simulink model "model2"  (R2020a)
settings: Solver=VariableStepAuto  StartTime=0.0  StopTime=50  RelTol=1e-3
libraries: SignalEditorBlockLib x1
settings Model: Creator=MILAD  LastModifiedBy=payagostar
settings DataIOCC: ReturnWorkspaceOutputs=off
settings DebuggingCC: ArithmeticOperatorsInVariantConditions=warning
settings SFSimCC: CustomCodeUndefinedFunction=UseInterfaceOnly

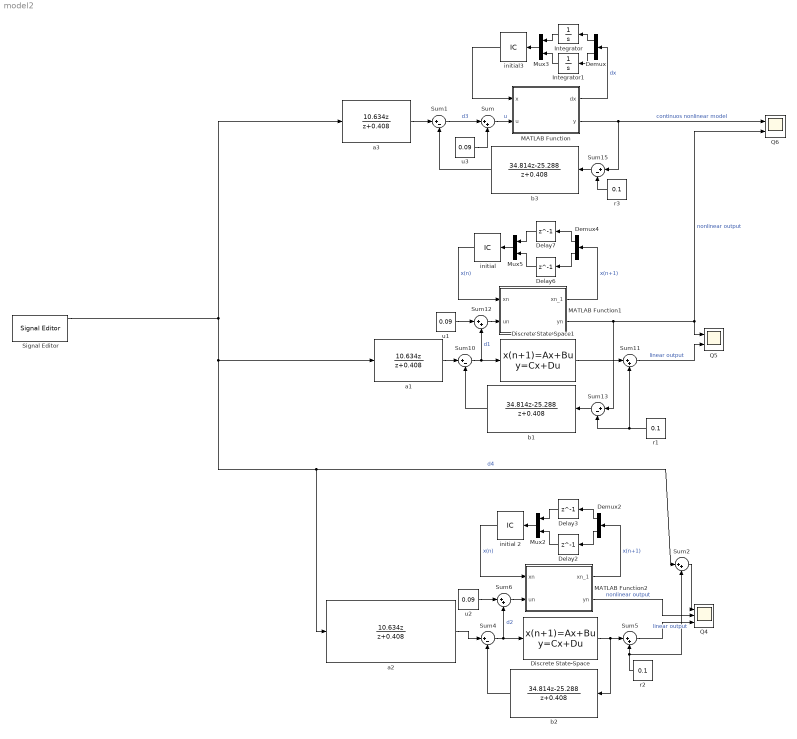
== system model2 ==
  " Q4" : Scope  NumInputPorts=3
  Delay{2..3,6..7} (4 alike) : Delay  DelayLength=1  InitialCondition=0  SampleTime=0.166
  Demux : Demux  Outputs=2
  Demux2 : Demux  Outputs=2
  Demux4 : Demux  Outputs=2
  Discrete State-Space : DiscreteStateSpace  A=[0.9884 0.1523;-0.1354 0.8361]  B=[0.01447;0.1693]  C=[1 0]  D=0  SampleTime=0.166
  Discrete State-Space1 : DiscreteStateSpace  A=[0.9884 0.1523;-0.1354 0.8361]  B=[0.01447;0.1693]  C=[1 0]  D=0  SampleTime=0.166
  Integrator : Integrator  InitialCondition=0.1
  Integrator1 : Integrator
  MATLAB Function : MATLAB Function  TreatAsAtomicUnit=on
  MATLAB Function1 : MATLAB Function  TreatAsAtomicUnit=on
  MATLAB Function2 : MATLAB Function  TreatAsAtomicUnit=on
  Mux2 : Mux  Inputs=2
  Mux3 : Mux  Inputs=2
  Mux5 : Mux  Inputs=2
  Q5 : Scope  NumInputPorts=2
  Q6 : Scope  NumInputPorts=2
  Signal Editor : SignalEditorBlockLib/Signal Editor  FileName=r.mat  ActiveScenario=Scenario  ActiveSignal=Signal 3  IsBus=off  OutputBusObjectStr=Bus: BusObject  SampleTime=0.166  Interpolate=off  ZeroCross=off  OutputAfterFinalValue=Setting to zero  Unit=inherit  PreserveSignalName=on
  Sum{,2,5..6,11..12} (6 alike) : Sum  Inputs=|++
  Sum{1,4,10,13,15} (5 alike) : Sum  Inputs=|+-
  a1 : DiscreteTransferFcn  Numerator=[10.634 0]  Denominator=[1, 0.408]  SampleTime=0.166
  a2 : DiscreteTransferFcn  Numerator=[10.634 0]  Denominator=[1 0.408]  SampleTime=0.166
  a3 : DiscreteTransferFcn  Numerator=[10.634 0]  Denominator=[1, 0.408]  SampleTime=0.166
  b1 : DiscreteTransferFcn  Numerator=[34.814 -25.288]  Denominator=[1, 0.408]  SampleTime=0.166
  b2 : DiscreteTransferFcn  Numerator=[34.814, -25.288]  Denominator=[1, 0.408]  SampleTime=0.166
  b3 : DiscreteTransferFcn  Numerator=[34.814, -25.288]  Denominator=[1, 0.408]  SampleTime=0.166
  initial : InitialCondition  Value=[0.1;0]
  initial 2 : InitialCondition  Value=[0.1;0]
  initial3 : InitialCondition  Value=[0.1;0]
  r1 : Constant  Value=0.1  SampleTime=0.166
  r2 : Constant  Value=0.1  SampleTime=0.166
  r3 : Constant  Value=0.1  SampleTime=0.166
  u1 : Constant  Value=0.09  SampleTime=0.166
  u2 : Constant  Value=0.09  SampleTime=0.166
  u3 : Constant  Value=0.09  SampleTime=0.166
  wires:
  Integrator1/1 -> Mux3/2
  Demux/1 -> Integrator/1
  Integrator/1 -> Mux3/1
  Mux3/1 -> initial3/1
  Demux/2 -> Integrator1/1
  u3/1 -> Sum/2
  initial3/1 -> MATLAB Function/1(x)
  Sum/1 -> MATLAB Function/2(u)  "u"
  MATLAB Function/1(dx) -> Demux/1  "dx"
  a2/1 -> Sum4/1
  b2/1 -> Sum4/2
  Sum4/1 -> Sum6/2, Discrete State-Space/1  "d2"
  Discrete State-Space/1 -> b2/1, Sum5/1
  initial 2/1 -> MATLAB Function2/1(xn)  "x(n)"
  Delay2/1 -> Mux2/2
  Demux2/2 -> Delay2/1
  Mux2/1 -> initial 2/1
  Delay3/1 -> Mux2/1
  Demux2/1 -> Delay3/1
  MATLAB Function2/1(xn_1) -> Demux2/1  "x(n+1)"
  MATLAB Function2/2(yn) -> " Q4"/2  "nonlinear output"
  u2/1 -> Sum6/1
  Sum6/1 -> MATLAB Function2/2(un)
  Sum5/1 -> " Q4"/3  "linear output"
  r2/1 -> Sum2/2, Sum5/2
  Signal Editor/1 -> Sum2/1, a2/1, a1/1, a3/1  "d4"
  a1/1 -> Sum10/1
  Sum12/1 -> MATLAB Function1/2(un)
  Discrete State-Space1/1 -> Sum11/1
  MATLAB Function1/2(yn) -> Sum13/1, Q6/2, Q5/1  "nonlinear output"
  u1/1 -> Sum12/1
  Delay7/1 -> Mux5/1
  b1/1 -> Sum10/2
  Demux4/2 -> Delay6/1
  Sum11/1 -> Q5/2  "linear output"
  initial/1 -> MATLAB Function1/1(xn)  "x(n)"
  Mux5/1 -> initial/1
  r1/1 -> Sum11/2, Sum13/2
  Demux4/1 -> Delay7/1
  MATLAB Function1/1(xn_1) -> Demux4/1  "x(n+1)"
  Sum10/1 -> Discrete State-Space1/1, Sum12/2  "d1"
  Delay6/1 -> Mux5/2
  Sum13/1 -> b1/1
  Sum1/1 -> Sum/1  "d3"
  r3/1 -> Sum15/2
  b3/1 -> Sum1/2
  Sum15/1 -> b3/1
  a3/1 -> Sum1/1
  MATLAB Function/2(y) -> Sum15/1, Q6/1  "continuos nonlinear model"
  Sum2/1 -> " Q4"/1

== matlab function model2/MATLAB Function1 ==
  data: xn input; xn_1 output; un input; yn output
function [xn_1,yn] = g1(xn,un)
xn_1 = [xn(1)+0.166*xn(2);-0.166*xn(1)+(1-0.166)*xn(2)+0.166*un/(1-xn(1))];
yn = [1 0]*xn;

== matlab function model2/MATLAB Function ==
  data: x input; dx output; u input; y output
function [dx,y] = system(x,u)
dx = [x(2);-x(1)-x(2)+u/(1-x(1))];
y  = [1 0]*x;

== matlab function model2/MATLAB Function2 ==
  data: xn input; xn_1 output; un input; yn output
function [xn_1,yn] = g1(xn,un)
xn_1 = [xn(1)+0.166*xn(2);-0.166*xn(1)+(1-0.166)*xn(2)+0.166*un/(1-xn(1))];
yn = [1 0]*xn;
